simulink model "Pendulum_LP"  (R2024a)
settings: Solver=FixedStepAuto  StartTime=0.0  StopTime=30  FixedStep=0.001  RelTol=1e-3
undefined symbols (not defined in the file): P1, P2, P3, P4, P5, P6, phi_dot_dot_sat, phi_dot_dot_threshold, tau_a_sat, tau_a_threshold, theta_dot_dot_sat, theta_dot_dot_threshold
settings Model: Creator=sipak  LastModifiedBy=sipak

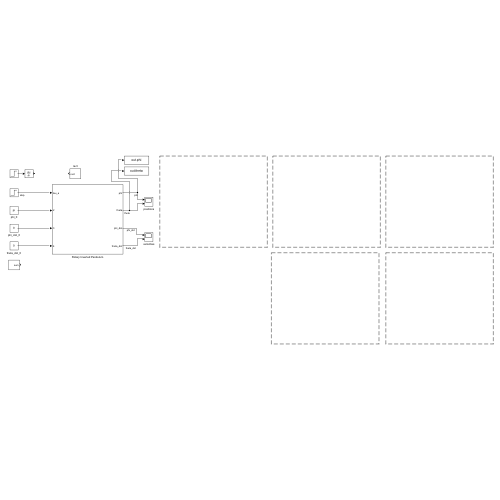
[thumbnail: Simulink's stored preview of the top-level diagram]
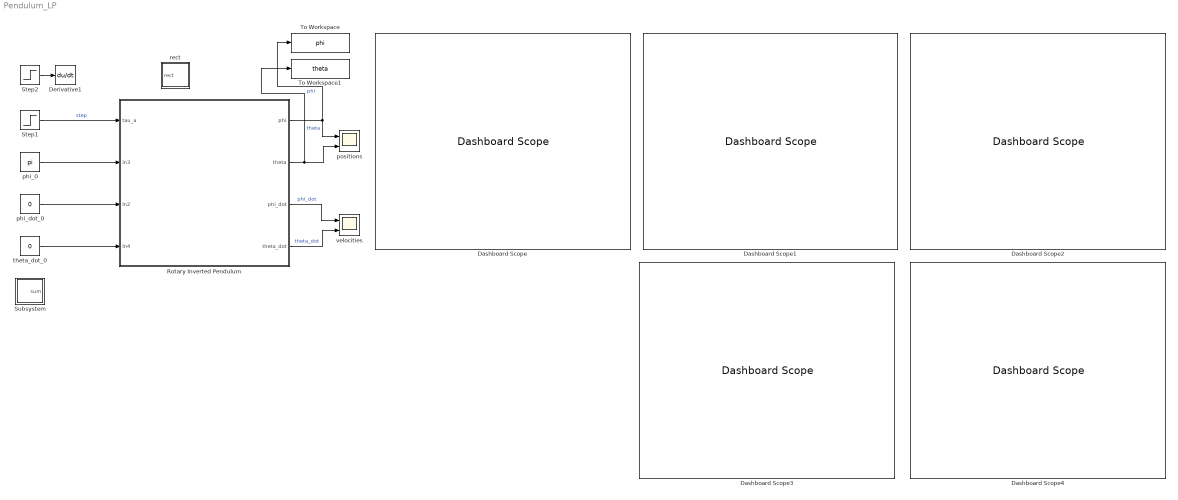
== system Pendulum_LP ==
  Dashboard Scope{,1..4} (5 alike) : DashboardScope
  Derivative1 : Derivative
  Rotary Inverted Pendulum : Subsystem
  Step1 : Step  After=10  SampleTime=0
  Step2 : Step  After=1e10  SampleTime=0
  Subsystem : Subsystem
  To Workspace : ToWorkspace  VariableName=phi  SampleTime=-1
      settings: Save2DSignal=2-D array (concatenate along first dimension)
  To Workspace1 : ToWorkspace  VariableName=theta  SampleTime=-1
      settings: Save2DSignal=2-D array (concatenate along first dimension)
  phi_0 : Constant  Value=pi
  phi_dot_0 : Constant  Value=0
  positions : Scope  NumInputPorts=2
  rect : Subsystem
  theta_dot_0 : Constant  Value=0
  velocities : Scope  NumInputPorts=2
  wires:
  phi_dot_0/1 -> Rotary Inverted Pendulum/3(In2)
  Rotary Inverted Pendulum/2(theta) -> To Workspace1/1, positions/2  "theta"
  Rotary Inverted Pendulum/1(phi) -> To Workspace/1, positions/1  "phi"
  phi_0/1 -> Rotary Inverted Pendulum/2(In3)
  Rotary Inverted Pendulum/3(phi_dot) -> velocities/1  "phi_dot"
  Rotary Inverted Pendulum/4(theta_dot) -> velocities/2  "theta_dot"
  theta_dot_0/1 -> Rotary Inverted Pendulum/4(In4)
  Step2/1 -> Derivative1/1
  Step1/1 -> Rotary Inverted Pendulum/1(tau_a)  "step"

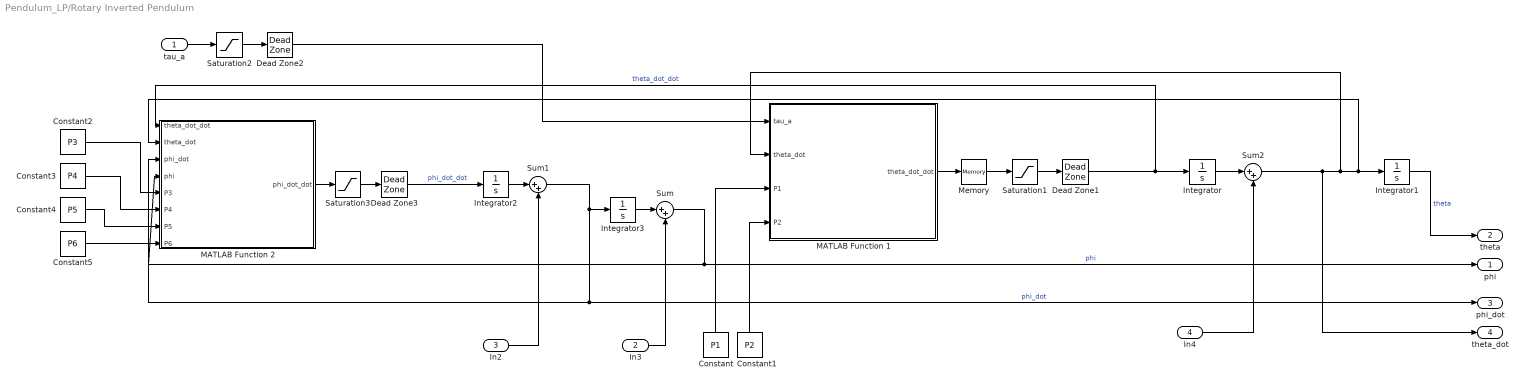
== system Pendulum_LP/Rotary Inverted Pendulum ==
  tau_a : Inport
  In3 : Inport  Port=2
  In2 : Inport  Port=3
  In4 : Inport  Port=4
  Constant : Constant  Value=P1
  Constant1 : Constant  Value=P2
  Constant2 : Constant  Value=P3
  Constant3 : Constant  Value=P4
  Constant4 : Constant  Value=P5
  Constant5 : Constant  Value=P6
  Dead Zone1 : DeadZone  LowerValue=-theta_dot_dot_threshold  UpperValue=theta_dot_dot_threshold
  Dead Zone2 : DeadZone  LowerValue=-tau_a_threshold  UpperValue=tau_a_threshold
  Dead Zone3 : DeadZone  LowerValue=-phi_dot_dot_threshold  UpperValue=phi_dot_dot_threshold
  Integrator{,1..3} (4 alike) : Integrator
  MATLAB Function 1 : MATLAB Function  TreatAsAtomicUnit=on
  MATLAB Function 2 : MATLAB Function  TreatAsAtomicUnit=on
  Memory : Memory
  Saturation1 : Saturate  UpperLimit=theta_dot_dot_sat  LowerLimit=-theta_dot_dot_sat
  Saturation2 : Saturate  UpperLimit=tau_a_sat  LowerLimit=-tau_a_sat
  Saturation3 : Saturate  UpperLimit=phi_dot_dot_sat  LowerLimit=-phi_dot_dot_sat
  Sum : Sum  Inputs=|++
  Sum1 : Sum  Inputs=|++
  Sum2 : Sum  Inputs=|++
  phi : Outport
  theta : Outport  Port=2
  phi_dot : Outport  Port=3
  theta_dot : Outport  Port=4
  wires:
  Integrator2/1 -> Sum1/1
  Integrator/1 -> Sum2/1
  Sum/1 -> phi/1, MATLAB Function 2/4(phi)  "phi"
  MATLAB Function 2/1(phi_dot_dot) -> Saturation3/1
  In3/1 -> Sum/2
  tau_a/1 -> Saturation2/1
  Integrator3/1 -> Sum/1
  In4/1 -> Sum2/2
  In2/1 -> Sum1/2
  MATLAB Function 1/1(theta_dot_dot) -> Memory/1
  Integrator1/1 -> theta/1  "theta"
  Memory/1 -> Saturation1/1
  Sum1/1 -> phi_dot/1, MATLAB Function 2/3(phi_dot), Integrator3/1  "phi_dot"
  Sum2/1 -> MATLAB Function 1/2(theta_dot), MATLAB Function 2/2(theta_dot), Integrator1/1, theta_dot/1
  Saturation2/1 -> Dead Zone2/1
  Dead Zone2/1 -> MATLAB Function 1/1(tau_a)
  Dead Zone3/1 -> Integrator2/1  "phi_dot_dot"
  Saturation3/1 -> Dead Zone3/1
  Saturation1/1 -> Dead Zone1/1
  Dead Zone1/1 -> MATLAB Function 2/1(theta_dot_dot), Integrator/1  "theta_dot_dot"
  Constant2/1 -> MATLAB Function 2/5(P3)
  Constant4/1 -> MATLAB Function 2/7(P5)
  Constant3/1 -> MATLAB Function 2/6(P4)
  Constant5/1 -> MATLAB Function 2/8(P6)
  Constant/1 -> MATLAB Function 1/3(P1)
  Constant1/1 -> MATLAB Function 1/4(P2)

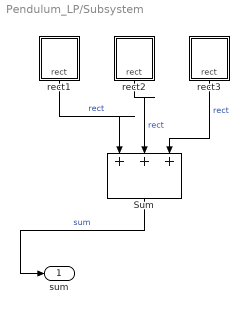
== system Pendulum_LP/Subsystem ==
  Sum : Sum  Inputs=|+++
  rect1 : Subsystem
  rect2 : Subsystem
  rect3 : Subsystem
  sum : Outport
  wires:
  Sum/1 -> sum/1  "sum"
  rect1/1(rect) -> Sum/1  "rect"
  rect2/1(rect) -> Sum/2  "rect"
  rect3/1(rect) -> Sum/3  "rect"

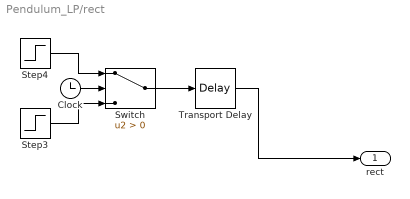
== system Pendulum_LP/rect ==
  Clock : Clock
  Step3 : Step  After=5  SampleTime=0
  Step4 : Step  Time=2  Before=5  After=0  SampleTime=0
  Switch : Switch  Criteria=u2 > Threshold  SaturateOnIntegerOverflow=off  InputSameDT=off
  Transport Delay : TransportDelay  DelayTime=0.3
  rect : Outport
  wires:
  Clock/1 -> Switch/2
  Step3/1 -> Switch/3
  Switch/1 -> Transport Delay/1
  Step4/1 -> Switch/1
  Transport Delay/1 -> rect/1

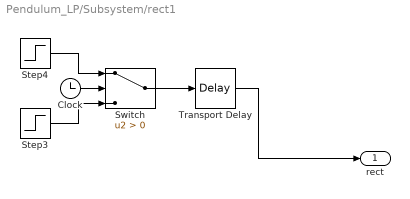
== system Pendulum_LP/Subsystem/rect1 ==
  Clock : Clock
  Step3 : Step  After=5  SampleTime=0
  Step4 : Step  Time=2  Before=5  After=0  SampleTime=0
  Switch : Switch  Criteria=u2 > Threshold  SaturateOnIntegerOverflow=off  InputSameDT=off
  Transport Delay : TransportDelay
  rect : Outport
  wires:
  Transport Delay/1 -> rect/1
  Step4/1 -> Switch/1
  Switch/1 -> Transport Delay/1
  Step3/1 -> Switch/3
  Clock/1 -> Switch/2

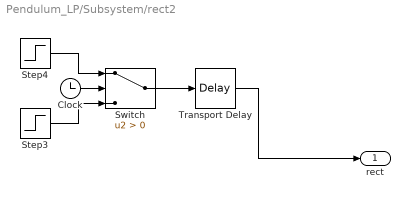
== system Pendulum_LP/Subsystem/rect2 ==
  Clock : Clock
  Step3 : Step  After=-5  SampleTime=0
  Step4 : Step  Time=2  Before=-5  After=0  SampleTime=0
  Switch : Switch  Criteria=u2 > Threshold  SaturateOnIntegerOverflow=off  InputSameDT=off
  Transport Delay : TransportDelay  DelayTime=4
  rect : Outport
  wires:
  Clock/1 -> Switch/2
  Step3/1 -> Switch/3
  Switch/1 -> Transport Delay/1
  Step4/1 -> Switch/1
  Transport Delay/1 -> rect/1

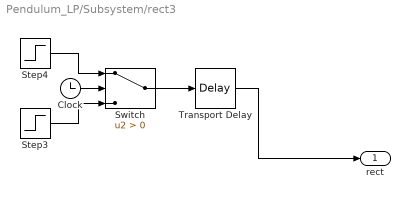
== system Pendulum_LP/Subsystem/rect3 ==
  Clock : Clock
  Step3 : Step  After=5  SampleTime=0
  Step4 : Step  Time=2  Before=5  After=0  SampleTime=0
  Switch : Switch  Criteria=u2 > Threshold  SaturateOnIntegerOverflow=off  InputSameDT=off
  Transport Delay : TransportDelay  DelayTime=7
  rect : Outport
  wires:
  Transport Delay/1 -> rect/1
  Step4/1 -> Switch/1
  Switch/1 -> Transport Delay/1
  Step3/1 -> Switch/3
  Clock/1 -> Switch/2

== matlab function Pendulum_LP/Rotary Inverted Pendulum/MATLAB Function 2 ==
  data: theta_dot_dot input; phi_dot_dot output; theta_dot input; phi_dot input; phi input; P3 input; P4 input; P5 input; P6 input
function phi_dot_dot = equation2(theta_dot_dot, theta_dot, phi_dot, phi, P3, P4, P5, P6)

    tau_p = 0;
    phi_dot_dot = (2 * tau_p - (P3 * theta_dot_dot * cos(phi)) ...
                   + (0 * theta_dot^2 * sin(2 * phi)) ... % We put 0 times the rest because Ip_y2 disappear when linearizing. That might be false
                   + (P6 * sin(phi)) ...
                   - (P5 * phi_dot)) / P4;
end

== matlab function Pendulum_LP/Rotary Inverted Pendulum/MATLAB Function 1 ==
  data: tau_a input; theta_dot_dot output; theta_dot input; P1 input; P2 input
function theta_dot_dot = equation1(tau_a, theta_dot, P1, P2)

    theta_dot_dot = (tau_a - (P2 * theta_dot)) / P1;
    
end
